simulink model "model_pid"  (R2013a)
settings: Solver=ode45  StartTime=0.0  StopTime=10.0  MaxStep=0.01  RelTol=1e-3
values from neighbouring files (symbols this model uses):
  Td = 1.5    [skrypt_pid.m]
  Tp = 0.1    [skrypt_pid.m]
  x = 0    [skrypt_pid.m]
undefined symbols (not defined in the file or in its folder): kr
settings Model: Creator=L13-4  LastModifiedBy=Dawid Perdek
settings DataIOCC: SignalLoggingSaveFormat=ModelDataLogs
settings DebuggingCC: UnderspecifiedInitializationDetection=Simplified  MultiTaskDSMMsg=warning  MultiTaskCondExecSysMsg=none  StateNameClashWarn=none  StrictBusMsg=ErrorOnBusTreatedAsVector
settings RTWCC: IncludeERTFirstTime=on
settings GRTTargetCC: CodeReplacementLibrary=None  CPPClassGenCompliant=on

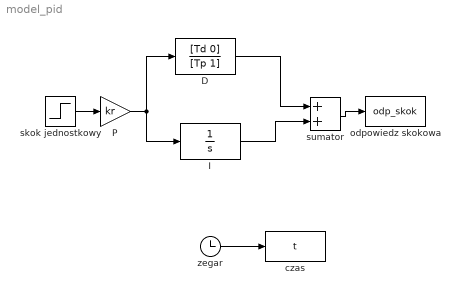
== system model_pid ==
  D : TransferFcn  Numerator=[Td 0]  Denominator=[Tp 1]
  I : TransferFcn  Numerator=[ 1 ]  Denominator=[1 0]
  P : Gain  Gain=kr
  czas : ToWorkspace  VariableName=t  SampleTime=-1
  odpowiedz skokowa : ToWorkspace  VariableName=odp_skok  SampleTime=-1
  skok jednostkowy : Step  Time=x  SampleTime=0
  sumator : Sum
  zegar : Clock
  wires:
  skok jednostkowy/1 -> P/1
  sumator/1 -> odpowiedz skokowa/1
  zegar/1 -> czas/1
  I/1 -> sumator/2
  P/1 -> I/1, D/1
  D/1 -> sumator/1
